simulink model "P7SLink"  (R2026a)
settings: Solver=VariableStepAuto  StopTime=5
values from neighbouring files (symbols this model uses):
  b = 0.0012    [P7Mat.m]
  J = 0.001    [P7Mat.m]
  Ke = 0.01    [P7Mat.m]
  Kt = 0.01    [P7Mat.m]
  La = 0.023    [P7Mat.m]
  Ra = 2    [P7Mat.m]

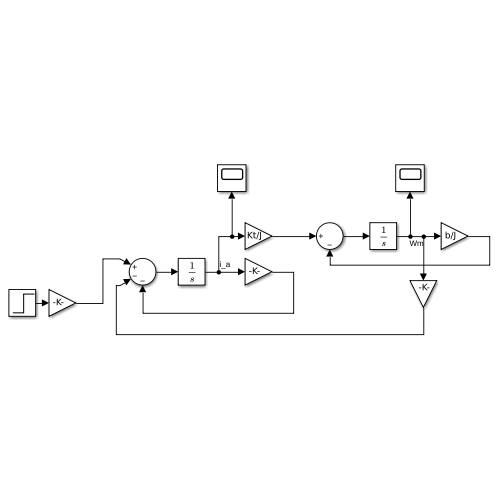
[thumbnail: Simulink's stored preview of the top-level diagram]
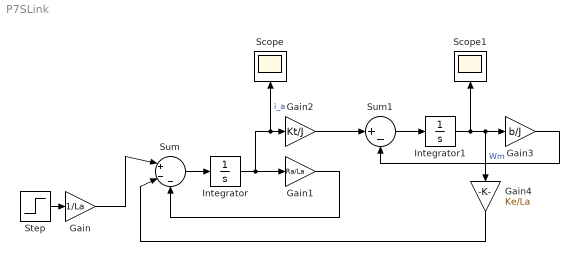
== system P7SLink ==
  Gain : Gain  Gain=1/La
  Gain1 : Gain  Gain=Ra/La
  Gain2 : Gain  Gain=Kt/J
  Gain3 : Gain  Gain=b/J
  Gain4 : Gain  Gain=Ke/La
  Integrator : Integrator
  Integrator1 : Integrator
  Scope : Scope
      settings: ActiveDisplayYMinimum=-0.31135315049383205  ActiveDisplayYMaximum=2.8021783544444889
  Scope1 : Scope
      settings: ActiveDisplayYMinimum=-2.4951237985135206  ActiveDisplayYMaximum=22.45611418662169
  Step : Step  Time=0  FinalValue=5  SampleTime=0
  Sum : Sum  Inputs=|+--
  Sum1 : Sum  Inputs=|+-
  wires:
  Step/1 -> Gain/1
  Gain/1 -> Sum/1
  Sum/1 -> Integrator/1
  Integrator/1 -> Gain1/1, Scope/1, Gain2/1  "i_a"
  Gain1/1 -> Sum/3
  Gain2/1 -> Sum1/1
  Sum1/1 -> Integrator1/1
  Integrator1/1 -> Scope1/1, Gain4/1, Gain3/1  "Wm"
  Gain3/1 -> Sum1/2
  Gain4/1 -> Sum/2
